simulink model "simulation_projet_ana_signal"  (Simulink 7.9)
settings: Solver=ode45  StartTime=0.0  StopTime=Tsim  RelTol=1e-3
values from neighbouring files (symbols this model uses):
  F1 = 85*10^3    (= 85000)    [traitement_du_signal.m]
  F2 = 90*10^3    (= 90000)    [traitement_du_signal.m]
  F3 = 95*10^3    (= 95000)    [traitement_du_signal.m]
  F4 = 100*10^3    (= 100000)    [traitement_du_signal.m]
  F5 = 115*10^3    (= 115000)    [traitement_du_signal.m]
  F6 = 120*10^3    (= 120000)    [traitement_du_signal.m]
  Te = T/M    (= 0.0625)    [script_simulation.m]    (also in traitement_du_signal.m = 3.125e-06)
settings Model: Creator=ahamada  LastModifiedBy=ahamada

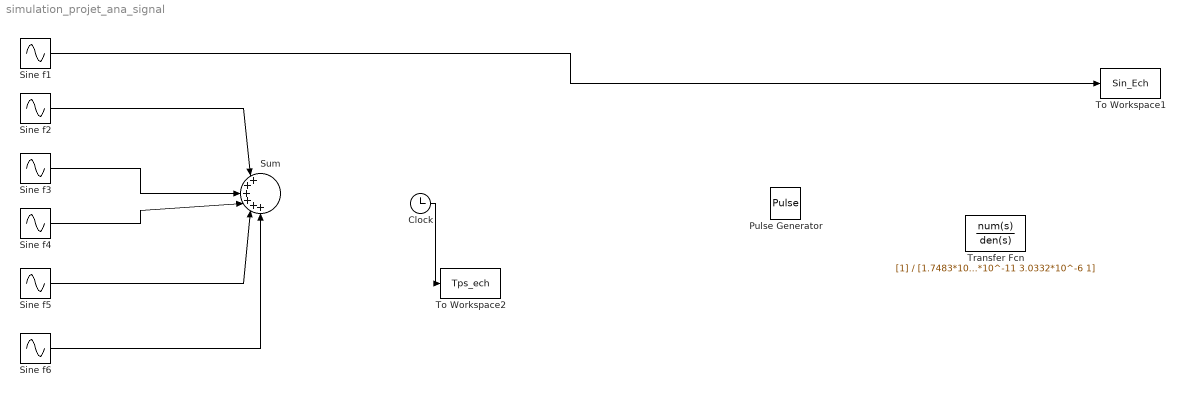
== system simulation_projet_ana_signal ==
  Clock : Clock
  Pulse Generator : DiscretePulseGenerator  PulseType=Time based  Period=1/F1  PulseWidth=50
  Sine f1 : Sin  Frequency=F1*2*pi  SampleTime=0
  Sine f2 : Sin  Frequency=F2*2*pi  SampleTime=0
  Sine f3 : Sin  Frequency=F3*2*pi  SampleTime=0
  Sine f4 : Sin  Frequency=F4*2*pi  SampleTime=0
  Sine f5 : Sin  Frequency=F5*2*pi  SampleTime=0
  Sine f6 : Sin  Frequency=F6*2*pi  SampleTime=0
  Sum : Sum  Inputs=|++++++
  To Workspace1 : ToWorkspace  VariableName=Sin_Ech  SampleTime=Te
  To Workspace2 : ToWorkspace  VariableName=Tps_ech  SampleTime=Te
  Transfer Fcn : TransferFcn  Denominator=[1.7483*10^-23 7.6663*10^-18 1.162*10^-11 3.0332*10^-6 1]
  wires:
  Clock/1 -> To Workspace2/1
  Sine f2/1 -> Sum/1
  Sine f3/1 -> Sum/3
  Sine f4/1 -> Sum/4
  Sine f5/1 -> Sum/5
  Sine f6/1 -> Sum/6
  Sine f1/1 -> To Workspace1/1
